simulink model "BFE_TestHarness"  (Simulink 8.6)
settings: Solver=FixedStepDiscrete  StartTime=0.0  StopTime=3  FixedStep=Ts  RelTol=1e-3
PreLoadFcn:
  | addpath('MBD_Tests')
  | 
  | load('Workspace\EnvVar.mat')
  | run('MBD_Tests\MBD_tests_init.m')
  | if exist('tl_preloadfcn','file'), tl_preloadfcn(gcs,402); end
PostLoadFcn:
  | if exist('tl_postloadfcn','file'), tl_postloadfcn(gcs,402); end
InitFcn:
  | if exist('tlds_init','file'), tlds_init(gcs); end
StartFcn:
  | if exist('tlds_start','file'), tlds_start(gcs); end
StopFcn:
  | if exist('tlds_stop','file'), tlds_stop(gcs); end
undefined symbols (not defined in the file): ddv, Ts, u2, u3, u4
libraries: tllib x11, simulink x8, LIB_TF_G_111 x2, LIB_TF_G_12_StepControl x2, LIB_TF_G_112 x1, LIB_TF_G_113 x1
(part 12 of 17)

== system BFE_TestHarness/BFE_AC_BeltFunctionExecution/Subsystem/BFE_AC_BeltFunctionExecution/BFE_AC_BeltFunctionExecution/BFE_runExecuteStandardSteps/ExecuteStandardSteps/SubsystemConvertOrderToMotorPower/RescaleOrderType/If Action Subsystem1 ==
  In1 : Inport
  Action Port : ActionPort  ActionType=else
  8Bit Decoder : Subsystem  RequirementInfo={} %GIDa_f55fd669_1c9c_4845_99fb_e2b5d961822e  mask(TLSAMPLES_8BIT_DECODER){}
      mask help:
      | Decodes one UInt8 byte into 8 bits.
      | All inputs are boolean variables.
      |
      | Sample implementation using TargetLink Custom Code block.
      | Version 1.0.
  Gain : Gain  RequirementInfo={} %GIDa_b55e4cd5_a38b_48ed_9505_573e117cd211  Gain=2  mask(TL_Gain){data={'output',{'type','UInt8'},'date',735951.66851049766}}
      settings: CopyFcn=if exist('tl_reset_reviewflag','file')==2,tl_reset_reviewflag(gcbh);end  DeleteFcn=if exist('delete_tlblock','file')==2,delete_tlblock(gcbh);end  NameChangeFcn=if exist('rename_tlblock','file')==2,rename_tlblock(gcbh);end  OpenFcn=if exist('tl_open_blockdlg','file')==2,tl_open_blockdlg(gcbh);else,open_system(gcbh,'parameter');end
      mask Help: eval(['if exist(''tl_online_help'',''file'') == 2, tl_online_help(''Topic'',''TL_Gain''),else, web([''jar:file:///'',matlabroot,''/help/toolbox/simulink/help.jar!/slref/' lower(get_param(gcbh,'Blocktype')) '.html''], ''-helpbrowser''),end'])
      mask Display: plot([0, .9, 0],[.05, .5, .95])
  Gain1 : Gain  RequirementInfo={} %GIDa_921c6136_ff97_4ffd_be38_728517461098  Gain=4  mask(TL_Gain){data={'output',{'type','UInt8'},'date',735951.6685099653}}
      settings: CopyFcn=if exist('tl_reset_reviewflag','file')==2,tl_reset_reviewflag(gcbh);end  DeleteFcn=if exist('delete_tlblock','file')==2,delete_tlblock(gcbh);end  NameChangeFcn=if exist('rename_tlblock','file')==2,rename_tlblock(gcbh);end  OpenFcn=if exist('tl_open_blockdlg','file')==2,tl_open_blockdlg(gcbh);else,open_system(gcbh,'parameter');end
      mask Help: eval(['if exist(''tl_online_help'',''file'') == 2, tl_online_help(''Topic'',''TL_Gain''),else, web([''jar:file:///'',matlabroot,''/help/toolbox/simulink/help.jar!/slref/' lower(get_param(gcbh,'Blocktype')) '.html''], ''-helpbrowser''),end'])
      mask Display: plot([0, .9, 0],[.05, .5, .95])
  KB_FALSE : Constant  RequirementInfo={} %GIDa_f915cd69_078a_4f01_913a_c107cac231ec  Value=ddv('BFE/KB_FALSE')  OutDataTypeStr=boolean  SampleTime=-1  mask(TL_Constant){data={'output',{'variable','BFE/KB_FALSE'},'date',735951.66850947915}}
      settings: CopyFcn=if exist('tl_reset_reviewflag','file')==2,tl_reset_reviewflag(gcbh);end  DeleteFcn=if exist('delete_tlblock','file')==2,delete_tlblock(gcbh);end  NameChangeFcn=if exist('rename_tlblock','file')==2,rename_tlblock(gcbh);end  OpenFcn=if exist('tl_open_blockdlg','file')==2,tl_open_blockdlg(gcbh);else,open_system(gcbh,'parameter');end
      mask Help: eval(['if exist(''tl_online_help'',''file'') == 2, tl_online_help(''Topic'',''TL_Constant''),else, web([''jar:file:///'',matlabroot,''/help/toolbox/simulink/help.jar!/slref/' lower(get_param(gcbh,'Blocktype')) '.html''], ''-helpbrowser''),end'])
      mask Display: plot([-0.05, 1.05, NaN, -0.05, 1.05],[.01, .01, NaN, .99, .99])
  Rescaler : DataTypeConversion  RequirementInfo={} %GIDa_ed10c978_5e72_47fc_a98c_eb1c5f44208f  OutDataTypeStr=boolean  SaturateOnIntegerOverflow=on  RndMeth=Zero  mask(TL_Rescaler){data={'output',{'type','Bool'},'date',735951.66850910883}}
      settings: DeleteFcn=if exist('delete_tlblock','file')==2,delete_tlblock(gcbh);end  NameChangeFcn=if exist('rename_tlblock','file')==2,rename_tlblock(gcbh);end  OpenFcn=if exist('tl_open_blockdlg','file')==2,tl_open_blockdlg(gcbh);else,open_system(gcbh,'parameter');end
      mask Help: eval(['if exist(''tl_online_help'',''file'') == 2, tl_online_help(''Topic'',''TL_Rescaler''),else, web([''jar:file:///'',matlabroot,''/help/toolbox/simulink/help.jar!/slref/' lower(get_param(gcbh,'Blocktype')) '.html''], ''-helpbrowser''),end'])
      mask Display: plot([-0.05, 1.05, NaN, -0.05, 1.05],[.01, .01, NaN, .99, .99])
  Rescaler1 : DataTypeConversion  RequirementInfo={} %GIDa_39b68c5d_5051_4b83_9c5f_930843829e5b  OutDataTypeStr=boolean  SaturateOnIntegerOverflow=on  RndMeth=Zero  mask(TL_Rescaler){data={'output',{'type','Bool'},'date',735951.66850879625}}
      settings: DeleteFcn=if exist('delete_tlblock','file')==2,delete_tlblock(gcbh);end  NameChangeFcn=if exist('rename_tlblock','file')==2,rename_tlblock(gcbh);end  OpenFcn=if exist('tl_open_blockdlg','file')==2,tl_open_blockdlg(gcbh);else,open_system(gcbh,'parameter');end
      mask Help: eval(['if exist(''tl_online_help'',''file'') == 2, tl_online_help(''Topic'',''TL_Rescaler''),else, web([''jar:file:///'',matlabroot,''/help/toolbox/simulink/help.jar!/slref/' lower(get_param(gcbh,'Blocktype')) '.html''], ''-helpbrowser''),end'])
      mask Display: plot([-0.05, 1.05, NaN, -0.05, 1.05],[.01, .01, NaN, .99, .99])
  Sum : Sum  RequirementInfo={} %GIDa_bf5901df_7e24_402b_87d5_4616e7e4f154  Inputs=+++  OutDataTypeStr=uint8  mask(TL_Sum){data={'output',{'type','UInt8'},'date',735951.66850847227}}
      settings: CopyFcn=if exist('tl_reset_reviewflag','file')==2,tl_reset_reviewflag(gcbh);end  DeleteFcn=if exist('delete_tlblock','file')==2,delete_tlblock(gcbh);end  NameChangeFcn=if exist('rename_tlblock','file')==2,rename_tlblock(gcbh);end  OpenFcn=if exist('tl_open_blockdlg','file')==2,tl_open_blockdlg(gcbh);else,open_system(gcbh,'parameter');end
      mask Help: eval(['if exist(''tl_online_help'',''file'') == 2, tl_online_help(''Topic'',''TL_Sum''),else, web([''jar:file:///'',matlabroot,''/help/toolbox/simulink/help.jar!/slref/' lower(get_param(gcbh,'Blocktype')) '.html''], ''-helpbrowser''),end'])
      mask Display: plot([-0.05, 1.05, NaN, -0.05, 1.05],[.01, .01, NaN, .99, .99])
  Terminator{,1..4} (5 alike) : Terminator
      Terminator settings: RequirementInfo={} %GIDa_b985a43b_a922_4bfa_a156_49d154a65af9
      Terminator1 settings: RequirementInfo={} %GIDa_fc42d90d_332d_43a2_90e4_e002a4ca21c9
      Terminator2 settings: RequirementInfo={} %GIDa_c30be6e3_f98f_4fdf_9aef_66184a0d9bee
      Terminator3 settings: RequirementInfo={} %GIDa_10c7749e_891f_45dd_8967_1645b4253ceb
      Terminator4 settings: RequirementInfo={} %GIDa_931308c7_6201_4a3e_a99a_b49a3b5d8f7f
  OrderType_Rescaled : Outport  RequirementInfo={} %GIDa_639f9323_bb74_44e0_b135_790af7847108  InitialOutput=7
  bIsPID_M : Outport  RequirementInfo={} %GIDa_516cba01_1310_449a_8ead_50a9a6e6e36d  Port=2  InitialOutput=0
  IsPID_S : Outport  RequirementInfo={} %GIDa_34f540e5_dbe7_4732_a14a_d7da8304fe8a  Port=3  InitialOutput=0
  wires:
  8Bit Decoder/1(Bit7) -> Terminator/1
  8Bit Decoder/2(Bit6) -> Terminator1/1
  8Bit Decoder/5(Bit3) -> Terminator2/1
  8Bit Decoder/6(Bit2) -> Gain1/1
  8Bit Decoder/7(Bit1) -> Gain/1
  Gain1/1 -> Sum/1
  Gain/1 -> Sum/2
  8Bit Decoder/8(Bit0) -> Sum/3
  In1/1 -> 8Bit Decoder/1(U8in)
  Sum/1 -> OrderType_Rescaled/1
  8Bit Decoder/3(Bit5) -> Terminator4/1
  8Bit Decoder/4(Bit4) -> Terminator3/1
  Rescaler/1 -> bIsPID_M/1
  Rescaler1/1 -> IsPID_S/1
  KB_FALSE/1 -> Rescaler/1, Rescaler1/1

== system BFE_TestHarness/BFE_AC_BeltFunctionExecution/Subsystem/BFE_AC_BeltFunctionExecution/BFE_AC_BeltFunctionExecution/BFE_runExecuteStandardSteps/ExecuteStandardSteps/Mange Power Stage consign update/Call PAL service to update the PWM/Apply power order/If Action Subsystem ==
  MotorPowerOrder : Inport  RequirementInfo={} %GIDa_8a3e0fab_6469_49d0_b0e7_3cc1aded27fb  OutDataTypeStr=int16
  BoostPowerOrder : Inport  RequirementInfo={} %GIDa_c62afe18_b8e8_4ba5_bec0_673a8fe82bb6  Port=2  OutDataTypeStr=int16
  Action Port : ActionPort  RequirementInfo={} %GIDa_dec1255b_3724_4d91_8955_da5b3082da1f  ActionType=then
  Data Store Write1 : DataStoreWrite  RequirementInfo={} %GIDa_d0d6fb00_a7d1_4def_9c5c_b6d36554e87c  DataStoreName=BoostPowerOrder  mask(TL_DataStoreWrite){data={'date',735951.66840413189}}
      settings: DeleteFcn=if exist('delete_tlblock','file')==2,delete_tlblock(gcbh);end  NameChangeFcn=if exist('rename_tlblock','file')==2,rename_tlblock(gcbh);end  OpenFcn=if exist('tl_open_blockdlg','file')==2,tl_open_blockdlg(gcbh);else,open_system(gcbh,'parameter');end
      mask Help: eval(['if exist(''tl_online_help'',''file'') == 2, tl_online_help(''Topic'',''TL_DataStoreWrite''),else, web([''jar:file:///'',matlabroot,''/help/toolbox/simulink/help.jar!/slref/' lower(get_param(gcbh,'Blocktype')) '.html''], ''-helpbrowser''),end'])
      mask Display: plot([-0.05, 1.05, NaN, -0.05, 1.05],[.01, .01, NaN, .99, .99])
  Data Store Write2 : DataStoreWrite  RequirementInfo={} %GIDa_e00dfc7a_29b6_4634_91ac_a8b115b9033d  DataStoreName=MotorPowerOrder  mask(TL_DataStoreWrite){data={'date',735951.66840402782}}
      settings: DeleteFcn=if exist('delete_tlblock','file')==2,delete_tlblock(gcbh);end  NameChangeFcn=if exist('rename_tlblock','file')==2,rename_tlblock(gcbh);end  OpenFcn=if exist('tl_open_blockdlg','file')==2,tl_open_blockdlg(gcbh);else,open_system(gcbh,'parameter');end
      mask Help: eval(['if exist(''tl_online_help'',''file'') == 2, tl_online_help(''Topic'',''TL_DataStoreWrite''),else, web([''jar:file:///'',matlabroot,''/help/toolbox/simulink/help.jar!/slref/' lower(get_param(gcbh,'Blocktype')) '.html''], ''-helpbrowser''),end'])
      mask Display: plot([-0.05, 1.05, NaN, -0.05, 1.05],[.01, .01, NaN, .99, .99])
  Data Type Conversion : DataTypeConversion
  wires:
  MotorPowerOrder/1 -> Data Store Write2/1
  BoostPowerOrder/1 -> Data Type Conversion/1
  Data Type Conversion/1 -> Data Store Write1/1

== system BFE_TestHarness/BFE_AC_BeltFunctionExecution/Subsystem/BFE_AC_BeltFunctionExecution/BFE_AC_BeltFunctionExecution/BFE_runExecuteStandardSteps/ExecuteStandardSteps/SubsystemConvertOrderToMotorPower/Current_Regulation/PID Regulation/PID feature disabled ==
  Action Port : ActionPort  ActionType=else
  Constant : Constant  RequirementInfo={} %GIDa_e4d6bd68_2685_46fa_8e20_8917170c5f59  Value=ddv('Common/KS16_ZERO')  OutDataTypeStr=int16  mask(TL_Constant){data={'output',{'variable','Common/KS16_ZERO'},'date',735951.66839365743}}
      settings: CopyFcn=if exist('tl_reset_reviewflag','file')==2,tl_reset_reviewflag(gcbh);end  DeleteFcn=if exist('delete_tlblock','file')==2,delete_tlblock(gcbh);end  NameChangeFcn=if exist('rename_tlblock','file')==2,rename_tlblock(gcbh);end  OpenFcn=if exist('tl_open_blockdlg','file')==2,tl_open_blockdlg(gcbh);else,open_system(gcbh,'parameter');end
      mask Help: eval(['if exist(''tl_online_help'',''file'') == 2, tl_online_help(''Topic'',''TL_Constant''),else, web([''jar:file:///'',matlabroot,''/help/toolbox/simulink/help.jar!/slref/' lower(get_param(gcbh,'Blocktype')) '.html''], ''-helpbrowser''),end'])
      mask Display: plot([-0.05, 1.05, NaN, -0.05, 1.05],[.01, .01, NaN, .99, .99])
  Constant4 : Constant  RequirementInfo={} %GIDa_e92d9a50_0792_40c1_87bb_ea616f947e08  Value=ddv('Common/KS32_ZERO')  OutDataTypeStr=int32  mask(TL_Constant){data={'output',{'variable','Common/KS32_ZERO'},'date',735951.66839327547}}
      settings: AttributesFormatString=0  CopyFcn=if exist('tl_reset_reviewflag','file')==2,tl_reset_reviewflag(gcbh);end  DeleteFcn=if exist('delete_tlblock','file')==2,delete_tlblock(gcbh);end  NameChangeFcn=if exist('rename_tlblock','file')==2,rename_tlblock(gcbh);end  OpenFcn=if exist('tl_open_blockdlg','file')==2,tl_open_blockdlg(gcbh);else,open_system(gcbh,'parameter');end
      mask Help: eval(['if exist(''tl_online_help'',''file'') == 2, tl_online_help(''Topic'',''TL_Constant''),else, web([''jar:file:///'',matlabroot,''/help/toolbox/simulink/help.jar!/slref/' lower(get_param(gcbh,'Blocktype')) '.html''], ''-helpbrowser''),end'])
      mask Display: plot([-0.05, 1.05, NaN, -0.05, 1.05],[.01, .01, NaN, .99, .99])
  s16UnsaturatedMotorPowerOrder : Outport  RequirementInfo={} %GIDa_6c807ec4_1ccd_4ec5_b947_ca6e3aaa0757  InitialOutput=0
  s32IntegerError : Outport  RequirementInfo={} %GIDa_2849b0ab_a0d8_44cd_8224_2f762b5a6034  Port=2  InitialOutput=0
  wires:
  Constant4/1 -> s32IntegerError/1
  Constant/1 -> s16UnsaturatedMotorPowerOrder/1
